simulink model "sRes_eta"  (R2018b)
settings: Solver=ode23tb  StartTime=0.0  StopTime=3  MaxStep=10e-6  RelTol=1e-4  EnableMultiTasking=on
libraries: powerlib x9
settings Model: SimulationMode=accelerator  Creator=Gong Linxiao  LastModifiedBy=vibra
settings DataIOCC: LimitDataPoints=on  SaveFormat=Array
settings OptimizationCC: LifeSpan=inf
settings DebuggingCC: SolverPrmCheckMsg=warning  SFUnexpectedBacktrackingDiag=warning  SFNoUnconditionalDefaultTransitionDiag=warning  SFExecutionAtInitializationDiag=none
settings HardwareCC: ProdBitPerPointer=32  ProdBitPerSizeT=32  ProdBitPerPtrDiffT=32  ProdLargestAtomicFloat=None  ProdIntDivRoundTo=Undefined  ProdEndianess=Unspecified  ProdWordSize=32  ProdHWDeviceType=32-bit Generic
settings ModelReferenceCC: PropagateSignalLabelsOutOfModel=off
settings SFSimCC: SimUseLocalCustomCode=off
settings RTWCC: RTWUseLocalCustomCode=off
settings CodeAppCC: StateflowObjectComments=on
settings GRTTargetCC: TargetLangStandard=C89/C90 (ANSI)  GeneratePreprocessorConditionals=Disable all
settings ConfigComp: CovMetricSettings=dw  CovHtmlReporting=on  CovSaveCumulativeToWorkspaceVar=on  CovSaveSingleToWorkspaceVar=on  CovExternalEMLEnable=off  CovSFcnEnable=off
settings SimscapeCC: SimscapeNormalizeSystem=off

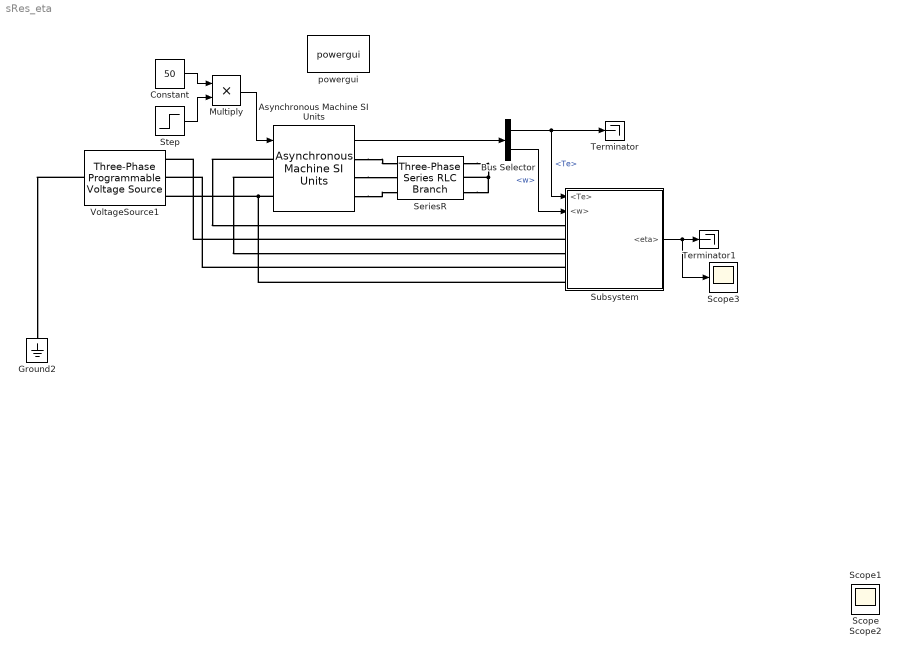
== system sRes_eta ==
  Asynchronous Machine SI Units : powerlib/Machines/Asynchronous Machine SI Units  RotorType=Wound  PresetModel="15:  5.4 HP (4KW)   400 V  50Hz 1430 RPM"  MechanicalLoad=Torque Tm  ShowDetailedParameters=on  ReferenceFrame=Stationary  Units=SI  MeasurementBus=on  NominalParameters=[4000 400 50]  Stator=[1.405 0.005839]  Rotor=[1.395 0.005839]  Cage1=[ 0.022 0.226/377]  Cage2=[ 0.022 0.226/377]  Lm=0.1722  Mechanical=[0.0131 0.002985 2]  PolePairs=2  InitialConditions=[1 0 0 0 0 0 0 0]  SimulateSaturation=off  Saturation=[14.03593122, 27.81365428, 53.79336849, 72.68890987, 97.98006896, 148.6815601, 215.7428561, 302.9841135, 420.4778367 ; 230, 322, 414, 460, 506, 552, 598, 644, 690]  LoadFlowParameters=1492000  TsPowergui=0  TsBlock=-1  IterativeModel=Trapezoidal non iterative  IterativeDiscreteModel=Trapezoidal non iterative  Pmec=0
      settings: SourceProductName=Simscape Electrical
  Bus Selector : BusSelector  OutputSignals=Te,w
  Constant : Constant  Value=50
  Ground2 : powerlib/Elements/Ground  LConnTagsString=a
      settings: SourceProductName=Simscape Electrical
  Multiply : Product
  Scope{,1..3} (4 alike) : Scope
  SeriesR : powerlib/Elements/Three-Phase Series RLC Branch  LConnTagsString=A|B|C  RConnTagsString=A|B|C  BranchType=R  Resistance=4  Inductance=1e-3  Capacitance=1e-6  Measurements=None
  Step : Step  Time=0.5  SampleTime=0
  Subsystem : Subsystem
  Terminator : Terminator
  Terminator1 : Terminator
  VoltageSource1 : powerlib/Electrical Sources/Three-Phase Programmable Voltage Source  PositiveSequence=[400 0 50]  VariationEntity=None  VariationType=Table of time-amplitude pairs  VariationTypeAlt=Step  VariationStep=20  VariationRate=30  VariationMagnitude=0.3  VariationFrequency=2  VariationTiming=[1 5]  VariationPhaseA=off  Amplitudes=[1 0.8 1.2 1.0]  TimeValues=[0 0.1 0.15 0.2]  HarmonicGeneration=off  HarmonicA=[3 0.2 -25 0]  HarmonicB=[2 0.15 35 2]  Timing="[0.05  3]"  BusType=PV  Pref=0  Qref=0  Qmin=-inf  Qmax=inf
      settings: SourceProductName=Simscape Electrical
  powergui : powerlib/powergui  Priority=1  SimulationMode=Continuous  SampleTime=50e-6  frequency=60  Iterations=50  frequencyindice=50  Pbase=100e6  ErrMax=1e-4  UnitsV=kV  UnitsW=MW  buscounter=0  FunctionMessages=off  echomessages=off  EnableUseOfTLC=off  CurrentSourceSwitches=on  DisableSnubberDevices=off  DisableRonSwitches=off  DisableVfSwitches=off  DisplayEquations=off  SolverType=Tustin  Interpol=off  ExternalGateDelay=off  methode=off  Ts=0  x0status=blocks  SPID=off  SwTol=0  HookPort=off  RestoreLinks=warning  ResistiveCurrentMeasurement=off  Frange=[0:2:500]  Ylog=off  Xlog=on  ShowGrid=off  save=off  variable=ZData  structure=0  ZoomFFT=off  StartTime=0.0  cycles=1  DisplayStyle=1  fundamental=60  FreqAxis=off  MaxFrequency=1000  frequencyindicesteady=50  RmsSteady=2  display=off
  wires:
  Asynchronous Machine SI Units/1 -> Bus Selector/1
  Bus Selector/1 -> Subsystem/1(<Te>), Terminator/1  "<Te>"
  Subsystem/1(<eta>) -> Scope3/1, Terminator1/1
  Bus Selector/2 -> Subsystem/2(<w>)  "<w>"
  Constant/1 -> Multiply/1
  Step/1 -> Multiply/2
  Multiply/1 -> Asynchronous Machine SI Units/1
  connections:
  SeriesR/RConn1 -- SeriesR/RConn3 -- SeriesR/RConn2
  Asynchronous Machine SI Units/RConn1 -- SeriesR/LConn1
  Asynchronous Machine SI Units/RConn2 -- SeriesR/LConn2
  Asynchronous Machine SI Units/RConn3 -- SeriesR/LConn3
  Subsystem/LConn4 -- VoltageSource1/RConn2
  Asynchronous Machine SI Units/LConn2 -- Subsystem/LConn3
  VoltageSource1/LConn1 -- Ground2/LConn1
  Asynchronous Machine SI Units/LConn1 -- Subsystem/LConn1
  Asynchronous Machine SI Units/LConn3 -- Subsystem/LConn5 -- VoltageSource1/RConn3
  Subsystem/LConn2 -- VoltageSource1/RConn1

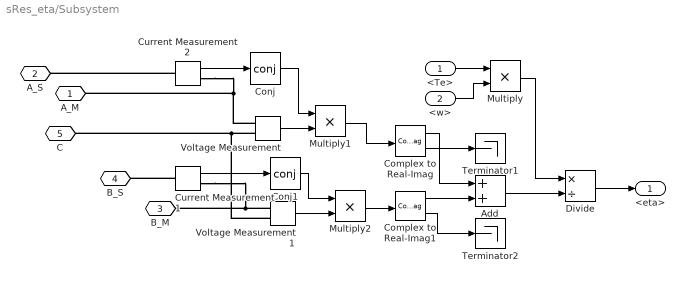
== system sRes_eta/Subsystem ==
  <Te> : Inport
  <w> : Inport  Port=2
  Add : Sum
  Complex to Real-Imag : ComplexToRealImag
  Complex to Real-Imag1 : ComplexToRealImag
  Conj : Math  Operator=conj  SaturateOnIntegerOverflow=on
  Conj1 : Math  Operator=conj  SaturateOnIntegerOverflow=on
  Current Measurement1 : powerlib/Measurements/Current Measurement  PhasorSimulation=off  OutputType=Complex  PSBequivalent=0
  Current Measurement2 : powerlib/Measurements/Current Measurement  PhasorSimulation=off  OutputType=Complex  PSBequivalent=0
  Divide : Product  Inputs=*/
  Multiply : Product
  Multiply1 : Product
  Multiply2 : Product
  Terminator1 : Terminator
  Terminator2 : Terminator
  Voltage Measurement : powerlib/Measurements/Voltage Measurement  PhasorSimulation=off  OutputType=Complex  PSBequivalent=0
  Voltage Measurement1 : powerlib/Measurements/Voltage Measurement  PhasorSimulation=off  OutputType=Complex  PSBequivalent=0
  A_M : PMIOPort  Side=Left
  A_S : PMIOPort  Port=2  Side=Left
  B_M : PMIOPort  Port=3  Side=Left
  B_S : PMIOPort  Port=4  Side=Left
  C : PMIOPort  Port=5  Side=Left
  <eta> : Outport
  wires:
  Complex to Real-Imag/2 -> Terminator1/1
  <w>/1 -> Multiply/2
  Complex to Real-Imag1/2 -> Terminator2/1
  Complex to Real-Imag/1 -> Add/1
  Complex to Real-Imag1/1 -> Add/2
  Multiply2/1 -> Complex to Real-Imag1/1
  Conj1/1 -> Multiply2/1
  Voltage Measurement/1 -> Multiply1/2
  Add/1 -> Divide/2
  Conj/1 -> Multiply1/1
  Current Measurement2/1 -> Conj/1
  Multiply1/1 -> Complex to Real-Imag/1
  Current Measurement1/1 -> Conj1/1
  <Te>/1 -> Multiply/1
  Multiply/1 -> Divide/1
  Voltage Measurement1/1 -> Multiply2/2
  Divide/1 -> <eta>/1
  connections:
  Current Measurement2/LConn1 -- A_S/RConn1
  Current Measurement1/RConn1 -- B_M/RConn1 -- Voltage Measurement1/LConn1
  Current Measurement2/RConn1 -- A_M/RConn1 -- Voltage Measurement/LConn1
  Voltage Measurement/LConn2 -- Voltage Measurement1/LConn2 -- C/RConn1
  Current Measurement1/LConn1 -- B_S/RConn1
